simulink model "doc_compander"  (Simulink 5.0)
settings: Solver=ode45  StartTime=0.0  StopTime=80  RelTol=1e-3
undefined symbols (not defined in the file): sig, slcm
libraries: commsrccod2 x3, dspsrcs4 x1
settings Model: Creator=agaltman  LastModifiedBy=agaltman  SignalLoggingName=logsOut  BlockReductionOpt=off  BooleanDataType=off  ConditionalExecOptimization=on  ZeroCrossControl=UseLocalSettings  RTWMathFcnLibMatFile=iso_c_tmw.mat  RTWOptions="-aEnforceIntegerDowncast=1 -aFoldNonRolledExpr=1 -aInlineInvariantSignals=1 -aInlineParameters=0 -aLocalBlockOutputs=1 -aRollThreshold=5 -aRTWVerbose=1 -aGenerateReport=0 -aForceParamTrailComments=0 -aGenerateComments=1 -aIgnoreCustomStorageClasses=1 -aIncHierarchyInIds=0 -aMaxRTWIdLen=31 -aShowEliminatedStatements=0 -aReadOnly=0 -aIncDataTypeInIds=0 -aPrefixModelToSubsysFcnNames=1 -aInlinedPrmAccess=\"Literals\" -aGenerateFullHeader=1 -aIsPILTarget=0 -aLogVarNameModifier=\"rt_\" -aExtMode=0 -aExtModeTesting=0 -aExtModeTransport=\"tcpip\"  -aInlineParameters=0"

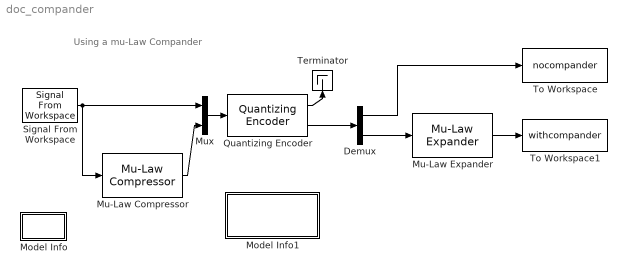
== system doc_compander ==
  note: Using a mu-Law Compander
  Demux : Demux  Outputs=2
  Model Info : Subsystem  LoadFcn=slcm LoadBlock;  InitFcn=slcm('UpdateAllCMBlocksInThisModelInit')  mask(CMBlock){InitialSaveTempField=, InitialBlockCM=none, BlockCM=none, Frame=on, SaveTempField=, DisplayStringWithTags=Info, MaskDisplayString=Info, HorizontalTextAlignment=Center, LeftAlignmentValue=0.5, SourceBlockDiagram=doc_compander, TagMaxNumber=20, CMTag1=, CMTag2=, CMTag3=, CMTag4=, CMTag5=, CMTag6=, CMTag7=, CMTag8=, CMTag9=, CMTag10=, CMTag11=, CMTag12=, CMTag13=, CMTag14=, CMTag15=, CMTag16=, CMTag17=, CMTag18=, CMTag19=, CMTag20=}
      mask help: This block allows revision control information to be displayed within the model.
      settings: CopyFcn=slcm CopyBlock;  DeleteFcn=slcm Cancel;  PostSaveFcn=slcm('UpdateAllCMBlocksInThisModel')  NameChangeFcn=slcm Rename;  OpenFcn=commdemohelp;
      mask Display: text(str2num(LeftAlignmentValue), 0.5, MaskDisplayString, 'HorizontalAlignment', HorizontalTextAlignment)
  Model Info1 : Subsystem  LoadFcn=slcm LoadBlock;  InitFcn=slcm('UpdateAllCMBlocksInThisModelInit')  mask(CMBlock){InitialSaveTempField=, InitialBlockCM=none, BlockCM=none, Frame=on, SaveTempField=, DisplayStringWithTags=Info, MaskDisplayString=Info, HorizontalTextAlignment=Center, LeftAlignmentValue=0.5, SourceBlockDiagram=doc_compander, TagMaxNumber=20, CMTag1=, CMTag2=, CMTag3=, CMTag4=, CMTag5=, CMTag6=, CMTag7=, CMTag8=, CMTag9=, CMTag10=, CMTag11=, CMTag12=, CMTag13=, CMTag14=, CMTag15=, CMTag16=, CMTag17=, CMTag18=, CMTag19=, CMTag20=}
      mask help: This block allows revision control information to be displayed within the model.
      settings: CopyFcn=slcm CopyBlock;  DeleteFcn=slcm Cancel;  PostSaveFcn=slcm('UpdateAllCMBlocksInThisModel')  NameChangeFcn=slcm Rename;  OpenFcn=sig = -4:.1:4; sig = exp(sig');
      mask Display: text(str2num(LeftAlignmentValue), 0.5, 'Double-click to\npreload data', 'HorizontalAlignment', HorizontalTextAlignment)
  Mu-Law Compressor : commsrccod2/Mu-Law Compressor  mu=255  V=max(sig)
  Mu-Law Expander : commsrccod2/Mu-Law Expander  mu=255  V=ceil(max(sig))
  Mux : Mux  Inputs=2
  Quantizing Encoder : commsrccod2/Quantizing Encoder  partition=0:floor(max(sig))  codebook=0:ceil(max(sig))
  Signal From Workspace : dspsrcs4/Signal From Workspace  X=sig  Ts=1  nsamps=1  OutputAfterFinalValue=Setting to zero
  Terminator : Terminator
      settings: Orientation=up
  To Workspace : ToWorkspace  VariableName=nocompander  SampleTime=-1  SaveFormat=Array
  To Workspace1 : ToWorkspace  VariableName=withcompander  SampleTime=-1  SaveFormat=Array
  wires:
  Signal From Workspace/1 -> Mux/1, Mu-Law Compressor/1
  Mu-Law Compressor/1 -> Mux/2
  Mux/1 -> Quantizing Encoder/1
  Quantizing Encoder/1 -> Terminator/1
  Quantizing Encoder/2 -> Demux/1
  Demux/2 -> Mu-Law Expander/1
  Mu-Law Expander/1 -> To Workspace1/1
  Demux/1 -> To Workspace/1

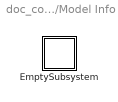
== system doc_compander/Model Info ==
  EmptySubsystem : Subsystem

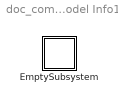
== system doc_compander/Model Info1 ==
  EmptySubsystem : Subsystem

== system doc_compander/Model Info/EmptySubsystem ==

== system doc_compander/Model Info1/EmptySubsystem ==
